simulink model "computervisionsimulation"  (R2019b)
settings: Solver=VariableStepDiscrete  StartTime=0.0  StopTime=1  RelTol=1e-3
undefined symbols (not defined in the file): gray, Rec, SDTV, strel
libraries: visionconversions x2, visionmorphops x2, visionfilter x1, visionsources x1, visiongeotforms x1
settings Model: Creator=DogukanArat  LastModifiedBy=DogukanArat

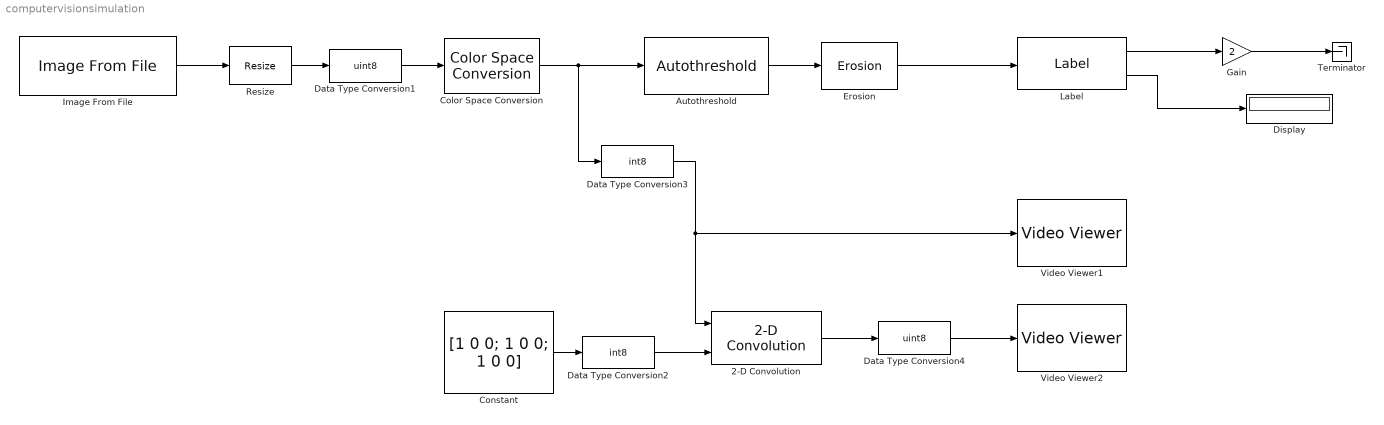
== system computervisionsimulation ==
  2-D Convolution : visionfilter/2-D Convolution  outSize=Same as input port I1  normalize=off  roundingMode=Floor  overflowMode=off  prodOutputMode=Binary point scaling  prodOutputWordLength=32  prodOutputFracLength=10  prodOutputSlope=0  accumSlope=2^-10  outputMode=Binary point scaling  outputWordLength=32  outputFracLength=12  outputSlope=2^-12
      settings: SourceProductName=Computer Vision Toolbox  SourceProductBaseCode=VP
  Autothreshold : visionconversions/Autothreshold  operator=>  threshOut=off  effMetricOut=off  userDefinedRange=off  umin=0  umax=255  outOfRngOpt=Ignore  scaleThreshold=off  scaleFactor=1  roundingMode=Floor  overflowMode=off  P1Mode=Specify word length  P1WordLength=32  P1FracLength=30  P1Slope=2^-30  A1Slope=2^-30  P2Mode=Specify word length  P2WordLength=32  P2FracLength=22  P2Slope=2^-22  A2Slope=2^-22  P3Mode=Specify word length  P3WordLength=32  P3FracLength=14  P3Slope=2^-14  A3Slope=2^-14  P4Mode=Binary point scaling  P4WordLength=32  P4FracLength=15  P4Slope=2^-15  A4Slope=2^-4  Q1Mode=Specify word length  Q1WordLength=32  Q1FracLength=16  Q1Slope=2^-16  EMMode=Specify word length  EMWordLength=16  EMFracLength=14  EMSlope=2^-14
      settings: SourceProductName=Computer Vision Toolbox  SourceProductBaseCode=VP
  Color Space Conversion : visionconversions/Color Space  Conversion  conversion=Obsolete  conversionActive=R'G'B' to intensity  wp_str=D65  rec=Rec. 601 (SDTV)  sys=1125/60/2:1  imagePorts=One multidimensional signal
  Constant : Constant  Value=[1 0 0; 1 0 0; 1 0 0]
  Data Type Conversion1 : DataTypeConversion  OutDataTypeStr=uint8
  Data Type Conversion2 : DataTypeConversion  OutDataTypeStr=int8
  Data Type Conversion3 : DataTypeConversion  OutDataTypeStr=int8
  Data Type Conversion4 : DataTypeConversion  OutDataTypeStr=uint8
  Display : Display
  Erosion : visionmorphops/Erosion  nhoodsrc=Specify via dialog  strel=strel('square',4)
      settings: SourceProductName=Computer Vision Toolbox  SourceProductBaseCode=VP
  Gain : Gain  Gain=2  OutDataTypeStr=uint8
  Image From File : visionsources/Image From File  Tag=vipblks_nd  FileName=D:\Github\smart-pill-box-embedded\src\resources\takenimage.jpg  Ts=inf  imagePorts=One multidimensional signal  OutPortLabels=R|G|B  ImageDataType=Inherit from input image  sdImageDataType=uint(8)  Signed=on  WordLength=16  FractionLengthMode=User-defined  FractionLength=15
      settings: SourceProductName=Computer Vision Toolbox
  Label : visionmorphops/Label  conn=8  output=Label matrix and number of labels  outType=Automatic  lastLabel=maximum value of the output data type
      settings: SourceProductName=Computer Vision Toolbox  SourceProductBaseCode=VP
  Resize : visiongeotforms/Resize  specify=Output size as a percentage of input size  rfactor=[20 20]  outCols=25  outRows=25  outRowsCols=[25 35]  interp_method=Bilinear  antialias=on  useROI=off  roiFlag=off  roundingMode=Nearest  overflowMode=on  prodOutputMode=Binary point scaling  prodOutputWordLength=32  prodOutputFracLength=10  prodOutputSlope=2^-10  accumSlope=2^-10  outputSlope=2^-10
      settings: SourceProductName=Computer Vision Toolbox  SourceProductBaseCode=VP
  Terminator : Terminator
  Video Viewer1 : VideoViewer  colormapValue=gray(256)  FigPos=[962 1037 958 929]  OpenAtMdlStart=off
  Video Viewer2 : VideoViewer  colormapValue=gray(256)  FigPos=[2 1037 958 929]  OpenAtMdlStart=off
  wires:
  Image From File/1 -> Resize/1
  Autothreshold/1 -> Erosion/1
  Erosion/1 -> Label/1
  Label/2 -> Display/1
  Label/1 -> Gain/1
  Gain/1 -> Terminator/1
  Resize/1 -> Data Type Conversion1/1
  Constant/1 -> Data Type Conversion2/1
  Data Type Conversion1/1 -> Color Space Conversion/1
  Data Type Conversion2/1 -> 2-D Convolution/2
  Color Space Conversion/1 -> Data Type Conversion3/1, Autothreshold/1
  2-D Convolution/1 -> Data Type Conversion4/1
  Data Type Conversion4/1 -> Video Viewer2/1
  Data Type Conversion3/1 -> Video Viewer1/1, 2-D Convolution/1
